simulink model "Q_onesml"  (R2021b)
settings: Solver=ode4  StartTime=0.0  StopTime=10  FixedStep=1e-3  RelTol=1e-3
StopFcn:
  | plot(out.tout,out.an.Data);
  | legend('Normal Acceleration');
  | grid;
  | 
  | figure;
  | plot(out.tout, out.q.Data);
  | legend('Pitch Rate')
  | grid;
values from neighbouring files (symbols this model uses):
  A = [0.4158,   1.025, -0.00267, -0.0001106, -0.080201,     0 ... (first row only)    [LQRExample.m]    (also in controllerdesingbig.m = A.A_implicit)
  B = [0 0;0 0;0 0;0 0;75 0;0 100]    [LQRExample.m]    (also in controllerdesingbig.m = B.B_implicit(:,4))
  C = [-1491, -146.43, -40.2, -0.9412, -1285, -564.66 ... (first row only)    [LQRExample.m]    (also in controllerdesingbig.m = [0.000000E+00, 1, 0.000000E+00, 0.000000E+00, 0.000000E+00, )
undefined symbols (not defined in the file or in its folder): K
settings Model: Creator=rfaie  LastModifiedBy=mo112

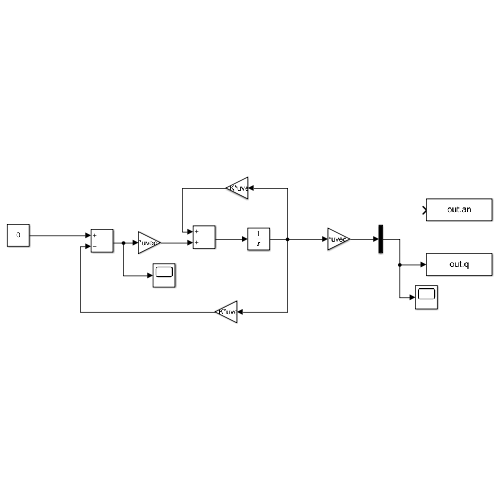
[thumbnail: Simulink's stored preview of the top-level diagram]
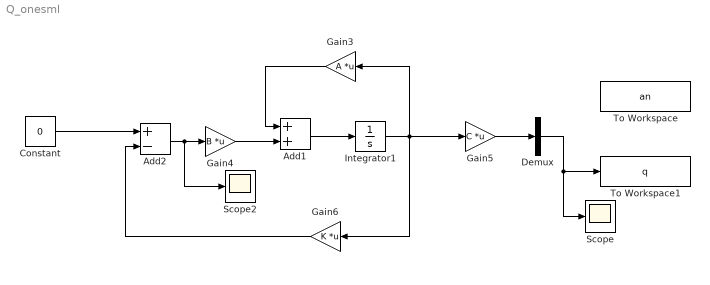
== system Q_onesml ==
  Add1 : Sum
  Add2 : Sum  Inputs=+-
  Constant : Constant  Value=0
  Demux : Demux  Outputs=1
  Gain3 : Gain  Gain=A  Multiplication=Matrix(K*u) (u vector)
  Gain4 : Gain  Gain=B  Multiplication=Matrix(K*u) (u vector)
  Gain5 : Gain  Gain=C  Multiplication=Matrix(K*u) (u vector)
  Gain6 : Gain  Gain=K  Multiplication=Matrix(K*u) (u vector)
  Integrator1 : Integrator  InitialCondition=[0, 0.2, 0]'
  Scope : Scope
  Scope2 : Scope
  To Workspace : ToWorkspace  VariableName=an  SaveFormat=Timeseries  SampleTime=-1
  To Workspace1 : ToWorkspace  VariableName=q  SaveFormat=Timeseries  SampleTime=-1
  wires:
  Gain3/1 -> Add1/1
  Add1/1 -> Integrator1/1
  Gain4/1 -> Add1/2
  Integrator1/1 -> Gain6/1, Gain3/1, Gain5/1
  Add2/1 -> Scope2/1, Gain4/1
  Constant/1 -> Add2/1
  Gain6/1 -> Add2/2
  Gain5/1 -> Demux/1
  Demux/1 -> To Workspace1/1, Scope/1
